simulink model "stilltesting2"  (R2017b)
settings: Solver=FixedStepAuto  StartTime=StartTime  StopTime=StopTime  FixedStep=StepSize  RelTol=1e-3
values from neighbouring files (symbols this model uses):
  a = a_d    (= 6782.423)    [AA279D_hw4.m]    (also in AA279D_hw4_v2.m = 7500; SCHAUBprop.m = oe(1); TLE_Reader.m = (mu/n^2)^(1/3); keplerUniversal.m = 1./alpha(idx))
  e = 0    [AA279D_PSET3.m]    (also in AA279D_PSET4.m = 0.1; AA279D_hw4.m = 0.7; AA279D_hw4_v2.m = 0.1; SCHAUBprop.m = oe(2))
  i = i_d    [AA279D_hw4.m]    (also in SCHAUBprop.m = oe(3); dv_hardcod.m = cin+1; dv_timer.m = cin+1; oe2roe.m = oe_c(3))
  M0 = M    [AA279D_FINAL.m]    (also in AA279D_PSET1.m; AA279D_PSET2.m; AA279D_PSET2_a_change.m; AA279D_PSET3.m)
  n = n_D    [AA279D_hw4.m]    (also in AA279D_hw4_v2.m = sqrt(mu/a^3); AA279D_hw5_dv.m = sqrt(mu/at^3); OE2ECI.m = sqrt(mu/a^3); TLE_Reader.m = revs_per_day*2*pi/(24*3600))
  Om = Om_d    [AA279D_hw4.m]    (also in SCHAUBprop.m = oe(4); oe2roe.m = oe_c(4); osc2mean.m = mod(Om, 2*pi) - (Om > pi)*2*pi)
  tol = 10^-5    (= 1e-05)    [AA279D_FINAL.m]    (also in AA279D_PSET1.m; AA279D_PSET2.m; AA279D_PSET2_a_change.m; AA279D_PSET3.m)
  w = 0    [AA279D_FINAL.m]    (also in AA279D_hw4.m = w_d; AA279D_hw4_v2.m = deg2rad(358.729); SCHAUBprop.m = oe(5); TLE_Reader.m = L3(1,6))
settings Model: Creator=Shawn Swist  LastModifiedBy=Shawn Swist

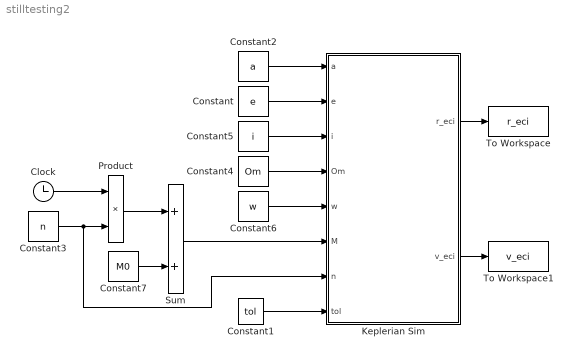
== system stilltesting2 ==
  Clock : Clock
  Constant : Constant  Value=e
  Constant1 : Constant  Value=tol
  Constant2 : Constant  Value=a
  Constant3 : Constant  Value=n
  Constant4 : Constant  Value=Om
  Constant5 : Constant  Value=i
  Constant6 : Constant  Value=w
  Constant7 : Constant  Value=M0
  Keplerian Sim : Subsystem
  Product : Product
  Sum : Sum
  To Workspace : ToWorkspace  VariableName=r_eci  SampleTime=-1
  To Workspace1 : ToWorkspace  VariableName=v_eci  SampleTime=-1
  wires:
  Constant3/1 -> Keplerian Sim/7(n), Product/2
  Clock/1 -> Product/1
  Product/1 -> Sum/1
  Constant7/1 -> Sum/2
  Constant/1 -> Keplerian Sim/2(e)
  Constant2/1 -> Keplerian Sim/1(a)
  Constant5/1 -> Keplerian Sim/3(i)
  Constant4/1 -> Keplerian Sim/4(Om)
  Constant6/1 -> Keplerian Sim/5(w)
  Constant1/1 -> Keplerian Sim/8(tol)
  Sum/1 -> Keplerian Sim/6(M)
  Keplerian Sim/2(v_eci) -> To Workspace1/1
  Keplerian Sim/1(r_eci) -> To Workspace/1

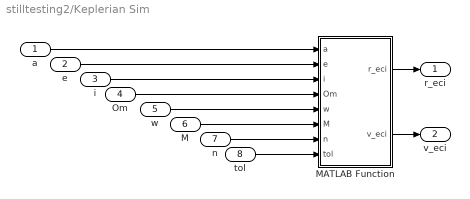
== system stilltesting2/Keplerian Sim ==
  a : Inport
  e : Inport  Port=2
  i : Inport  Port=3
  Om : Inport  Port=4
  w : Inport  Port=5
  M : Inport  Port=6
  n : Inport  Port=7
  tol : Inport  Port=8
  MATLAB Function : MATLAB Function  TreatAsAtomicUnit=on
  r_eci : Outport
  v_eci : Outport  Port=2
  wires:
  MATLAB Function/1(r_eci) -> r_eci/1
  MATLAB Function/2(v_eci) -> v_eci/1
  a/1 -> MATLAB Function/1(a)
  e/1 -> MATLAB Function/2(e)
  i/1 -> MATLAB Function/3(i)
  Om/1 -> MATLAB Function/4(Om)
  w/1 -> MATLAB Function/5(w)
  n/1 -> MATLAB Function/7(n)
  M/1 -> MATLAB Function/6(M)
  tol/1 -> MATLAB Function/8(tol)

== matlab function stilltesting2/Keplerian Sim/MATLAB Function ==
  data: a input; r_eci output; e input; i input; Om input; w input; M input; n input; v_eci output; tol input
function [r_eci, v_eci] = oe2eci(a,e,i,Om,w,M,n,tol)

% limit M
while M > 2*pi
    M = M -2*pi;
end

E = M2E(M, e, tol);    % rad

% Compute radius and velocity of orbit in perifocal coordinates
rPeri = [        a*(cos(E) - e);
         a*sqrt(1 - e^2)*sin(E);
                              0];

vPeriComp = [             -sin(E);
             sqrt(1 - e^2)*cos(E);
                                0];
vPeri = (a*n)/(1 - e*cos(E))*vPeriComp;

rotPeri2ECI = zeros(3,3);
% Develop rotation matrix depending on orbit shape/inclination
if i == 0 && e ~= 0         % Equatorial + elliptical
    rotPeri2ECI = rotz(rad2deg(w));
elseif e == 0 && i ~= 0     % Circular + inclined
    rotPeri2ECI = rotz(rad2deg(Om))*rotx(rad2deg(i));
elseif i == 0 && e == 0     % Equatorial + circular
    rotPeri2ECI = eye(3);
else                        % Elliptical + inclined
    rotPeri2ECI = rotz(rad2deg(Om))*rotx(rad2deg(i))*rotz(rad2deg(w));
end
    
% Rotate vectors into ECI frame
% r_eci = zeros(3,1);
% v_eci = zeros(3,1);
r_eci = rotPeri2ECI*rPeri;
v_eci = rotPeri2ECI*vPeri;

% r_eci = r_eci';
% v_eci = v_eci';
